simulink model "RL_TTS3_Controller_Blank"  (R2019b)
settings: Solver=FixedStepAuto  StartTime=0.0  StopTime=10.0  FixedStep=0.01  RelTol=1e-3
PostLoadFcn:
  | if any(exist('dsrtsu_mdlpostloadfcn', 'file') ~= 0), dsrtsu_mdlpostloadfcn('Execute', bdroot); end
undefined symbols (not defined in the file or in its folder): Ts
libraries: simulink x2
settings Model: DSRTSU_INTERNAL_RTI_VER=550  DSRTSU_INTERNAL_RTI_TYPE=rti1104  RTICANMMDATA=struct('GeneralSetupData',struct('modelroot','E:\Will\RemoteLabs\TTS3\HostPC','generalsettings',struct('filesettings',struct('destfolder',struct('Name','RTICANMM_FILES','Check',1),'buildfolder',struct('Name','.','Check',1),'AbsDestfolder',struct('Name','E:\Will\RemoteLabs\TTS3\HostPC\RTICANMM_FILES'),'AbsBuildfolder',struct('Name','E:\Will\RemoteLabs\TTS3\HostPC'))),'options',struct('addpaths',1,'rmpaths',1,'addtrcexclusion',true,'cannavigator',struct('checkmonitoring',0),'show_usrtrc',0,'use_usrtrc',0),'advanced',struct('options',ones(1,100)),'MPSetup',{{}},'RTI',struct('Type','RTI1104','Ver','7.13','Date','02-Nov-2019'),'modelname','TTS3_Controller_Test_OL','block','TTS3_Controller_Test_OL'))  DSRTSU_INTERNAL_RTIFPGA=150  Creator=whendrix  LastModifiedBy=edtve
settings DataIOCC: SaveOutput=off  SaveTime=off
settings OptimizationCC: BlockReduction=off  DefaultParameterBehavior=Inlined  OptimizeBlockIOStorage=off  BufferReuse=off  GlobalBufferReuse=off  ExpressionFolding=off  LocalBlockOutputs=off  OptimizeDataStoreBuffers=off  BusAssignmentInplaceUpdate=off
settings DebuggingCC: BusObjectLabelMismatch=none
settings HardwareCC: ProdBitPerPointer=32  ProdBitPerSizeT=32  ProdBitPerPtrDiffT=32  ProdLargestAtomicInteger=Integer  ProdEndianess=BigEndian  ProdWordSize=32  ProdHWDeviceType=Custom Processor->Custom  TargetIntDivRoundTo=Zero  TargetEndianess=BigEndian  TargetHWDeviceType=Custom Processor->Custom
settings ModelReferenceCC: ModelReferenceNumInstancesAllowed=Single  ModelReferenceMinAlgLoopOccurrences=on
settings SFSimCC: MATLABDynamicMemAlloc=off  CustomCodeUndefinedFunction=UseInterfaceOnly
settings RTWCC: Description=dSPACE DS1104 Hardware Platform  SystemTargetFile=rti1104.tlc  MakeCommand=make_rti  TemplateMakefile=rti1104.tmf
settings CodeAppCC: MaxIdLength=63
settings STFCustomTargetCC: ParMdlRefBuildCompliant=on  SystemTargetFile=rti1104.tlc
settings GRTTargetCC: TargetLangStandard=C89/C90 (ANSI)  CompOptLevelCompliant=off  ConcurrentExecutionCompliant=off  CombineOutputUpdateFcns=off  MatFileLogging=off  CPPClassGenCompliant=off  UseToolchainInfoCompliant=off

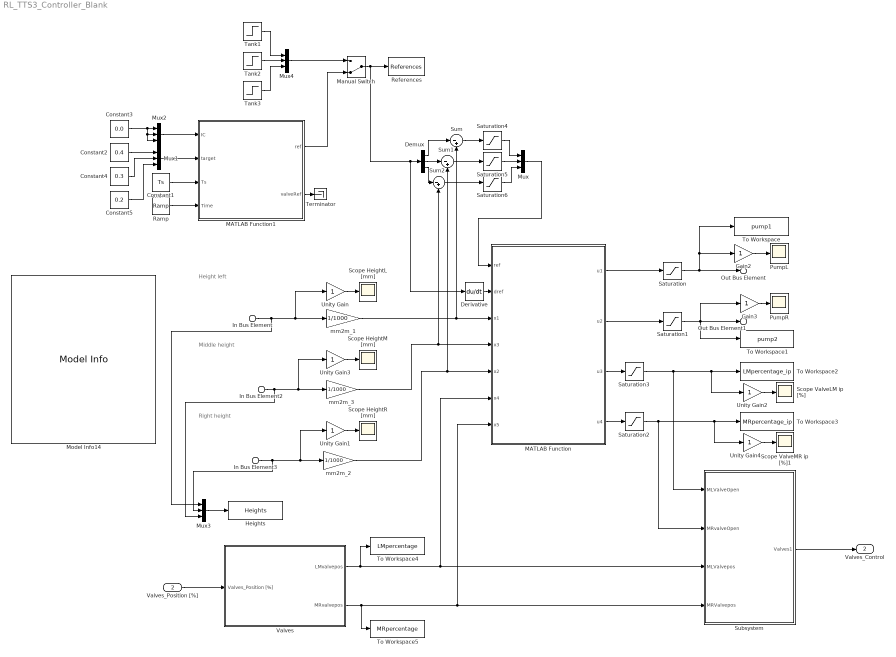
== system RL_TTS3_Controller_Blank ==
  note: Height left
  note: Middle height
  note: Right height
  In Bus Element : Inport  PortName=Heights [mm]  Element=Left
  In Bus Element2 : Inport  PortName=Heights [mm]  Element=Middle
  In Bus Element3 : Inport  PortName=Heights [mm]  Element=Right
  Valves_Position [%] : Inport  Port=2  OutDataTypeStr=Bus: ValvesSOCI
  Constant1 : Constant  Value=Ts
  Constant2 : Constant  Value=0.4
  Constant3 : Constant  Value=0.0
  Constant4 : Constant  Value=0.3
  Constant5 : Constant  Value=0.2
  Demux : Demux  Outputs=3
  Derivative : Derivative
  Gain2 : Gain
  Gain3 : Gain
  Heights : ToWorkspace  VariableName=Heights  SampleTime=-1
  MATLAB Function : MATLAB Function  TreatAsAtomicUnit=on
  MATLAB Function1 : MATLAB Function  TreatAsAtomicUnit=on
  Manual Switch : ManualSwitch  CurrentSetting=0
  Model Info14 : simulink/Model-Wide Utilities/Model Info  Frame=on  DisplayStringWithTags=|  HorizontalTextAlignment=Left  LeftAlignmentValue=0.02
      | Start model for the "Three Tank"
      | experiment on the "Three Tank" setup.
      | Version: 1.0
      | 
      | 
      | INFORMATION
      | ----------------------
      | 
      | Unity Gain block before Scope is needed for
      | RemoteLabs compatebility. 
      | Do not modify or remove!
      | 
      | Pump range:
      | 0 to 0.102 [l/s]
      | 
      | The 5 Valves are labeled according 
      | to their position:
      | 
      |    LM  MR
      |      X     X
      |  X      X      X
      | LD    MD   RD
      | 
      | L = Left
      | M = Middle
      | R = Right
      | D = Down
  Mux{,1..4} (5 alike) : Mux  Inputs=3
  PumpL : Scope
  "PumpR " : Scope
  Ramp : simulink/Sources/Ramp  slope=1  start=0  InitialOutput=0
  "References " : ToWorkspace  VariableName=References  SampleTime=-1
  Saturation : Saturate  UpperLimit=0.1  LowerLimit=0
  Saturation1 : Saturate  UpperLimit=0.1  LowerLimit=0
  Saturation2 : Saturate  UpperLimit=100  LowerLimit=0
  Saturation3 : Saturate  UpperLimit=100  LowerLimit=0
  Saturation4 : Saturate  UpperLimit=1  LowerLimit=-1
  Saturation5 : Saturate  UpperLimit=1  LowerLimit=-1
  Saturation6 : Saturate  UpperLimit=1  LowerLimit=-1
  Scope HeightL [mm] : Scope
  Scope HeightM [mm] : Scope
  Scope HeightR [mm] : Scope
  Scope ValveLM ip [%] : Scope
  Scope ValveMR ip [%]1 : Scope
  Subsystem : Subsystem
  Sum : Sum  Inputs=|-+
  Sum1 : Sum  Inputs=|-+
  Sum2 : Sum  Inputs=|-+
  Tank1 : Step  After=0.3  SampleTime=0
  Tank2 : Step  After=0.3  SampleTime=0
  Tank3 : Step  After=0.3  SampleTime=0
  Terminator : Terminator
  To Workspace : ToWorkspace  VariableName=pump1  SampleTime=-1
  To Workspace1 : ToWorkspace  VariableName=pump2  SampleTime=-1
  To Workspace2 : ToWorkspace  VariableName=LMpercentage_ip  SampleTime=-1
  To Workspace3 : ToWorkspace  VariableName=MRpercentage_ip  SampleTime=-1
  To Workspace4 : ToWorkspace  VariableName=LMpercentage  SampleTime=-1
  To Workspace5 : ToWorkspace  VariableName=MRpercentage  SampleTime=-1
  Unity Gain{,1..4} (5 alike) : Gain
  Valves : Subsystem  TreatAsAtomicUnit=on
  mm2m_1 : Gain  Gain=1/1000
  mm2m_2 : Gain  Gain=1/1000
  mm2m_3 : Gain  Gain=1/1000
  Out Bus Element : Outport  VectorParamsAs1DForOutWhenUnconnected=off  PortName=Pumps [l/s]  Element=Left
  Out Bus Element1 : Outport  VectorParamsAs1DForOutWhenUnconnected=off  PortName=Pumps [l/s]  Element=Right
  Valves_Control : Outport  Port=2  OutDataTypeStr=Bus: ValvesSICO  VectorParamsAs1DForOutWhenUnconnected=off
  wires:
  Unity Gain3/1 -> Scope HeightM [mm]/1
  Unity Gain1/1 -> Scope HeightR [mm]/1
  In Bus Element/1 -> Mux3/1, mm2m_1/1, Unity Gain/1
  In Bus Element2/1 -> Mux3/3, mm2m_3/1, Unity Gain3/1
  Valves_Position [%]/1 -> Valves/1(Valves_Position [%])
  Unity Gain/1 -> Scope HeightL [mm]/1
  Subsystem/1(Valves1) -> Valves_Control/1
  Valves/1(LMvalvepos) -> To Workspace4/1, MATLAB Function/6(x4), Subsystem/3(MLValvepos)
  Valves/2("MRvalvepos ") -> To Workspace5/1, MATLAB Function/7(x5), Subsystem/4(MRValvepos)
  Ramp/1 -> MATLAB Function1/4(Time)
  Constant1/1 -> MATLAB Function1/3(Ts)
  Constant2/1 -> Mux1/1
  Mux1/1 -> MATLAB Function1/2(target)
  Mux2/1 -> MATLAB Function1/1(IC)
  Constant3/1 -> Mux2/3, Mux2/2, Mux2/1
  MATLAB Function1/2(valveRef) -> Terminator/1
  mm2m_1/1 -> Sum/2, MATLAB Function/3(x1)
  mm2m_2/1 -> Sum1/2, MATLAB Function/5(x2)
  mm2m_3/1 -> Sum2/2, MATLAB Function/4(x3)
  MATLAB Function/4(u4) -> Saturation2/1
  MATLAB Function/3(u3) -> Saturation3/1
  Saturation3/1 -> Subsystem/1("MLValveOpen "), Unity Gain2/1, To Workspace2/1
  Saturation2/1 -> Subsystem/2(MRvalveOpen), Unity Gain4/1, To Workspace3/1
  Derivative/1 -> MATLAB Function/2(dref)
  In Bus Element3/1 -> mm2m_2/1, Unity Gain1/1, Mux3/2
  Mux3/1 -> Heights/1
  Tank2/1 -> Mux4/2
  Tank1/1 -> Mux4/1
  Tank3/1 -> Mux4/3
  MATLAB Function1/1(ref) -> Manual Switch/2
  Mux4/1 -> Manual Switch/1
  Manual Switch/1 -> "References "/1, Demux/1, Derivative/1
  Saturation/1 -> To Workspace/1, Gain2/1, Out Bus Element/1
  Saturation1/1 -> To Workspace1/1, Gain3/1, Out Bus Element1/1
  MATLAB Function/2(u2) -> Saturation1/1
  Gain3/1 -> "PumpR "/1
  Gain2/1 -> PumpL/1
  Demux/1 -> Sum/1
  Sum/1 -> Saturation4/1
  Demux/2 -> Sum1/1
  Sum1/1 -> Saturation5/1
  Demux/3 -> Sum2/1
  Sum2/1 -> Saturation6/1
  Saturation5/1 -> Mux/2
  Saturation4/1 -> Mux/1
  Saturation6/1 -> Mux/3
  Mux/1 -> MATLAB Function/1(ref)
  MATLAB Function/1(u1) -> Saturation/1
  Unity Gain2/1 -> Scope ValveLM ip [%]/1
  Unity Gain4/1 -> Scope ValveMR ip [%]1/1
  Constant4/1 -> Mux1/2
  Constant5/1 -> Mux1/3

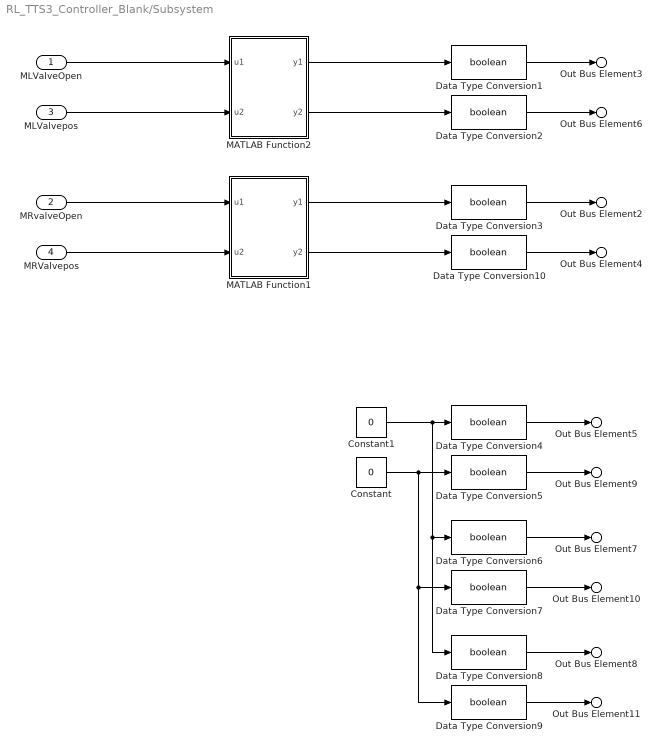
== system RL_TTS3_Controller_Blank/Subsystem ==
  "MLValveOpen " : Inport
  MRvalveOpen : Inport  Port=2
  MLValvepos : Inport  Port=3
  MRValvepos : Inport  Port=4
  Constant : Constant  Value=0
  Constant1 : Constant  Value=0
  Data Type Conversion{1..10} (10 alike) : DataTypeConversion  OutDataTypeStr=boolean
  MATLAB Function1 : MATLAB Function  TreatAsAtomicUnit=on
  MATLAB Function2 : MATLAB Function  TreatAsAtomicUnit=on
  Out Bus Element8 : Outport  VectorParamsAs1DForOutWhenUnconnected=off  PortName=Valves1  Element=RightDown.Open
  Out Bus Element11 : Outport  VectorParamsAs1DForOutWhenUnconnected=off  PortName=Valves1  Element=RightDown.Close
  Out Bus Element5 : Outport  VectorParamsAs1DForOutWhenUnconnected=off  PortName=Valves1  Element=LeftDown.Open
  Out Bus Element9 : Outport  VectorParamsAs1DForOutWhenUnconnected=off  PortName=Valves1  Element=LeftDown.Close
  Out Bus Element7 : Outport  VectorParamsAs1DForOutWhenUnconnected=off  PortName=Valves1  Element=MiddleDown.Open
  Out Bus Element10 : Outport  VectorParamsAs1DForOutWhenUnconnected=off  PortName=Valves1  Element=MiddleDown.Close
  Out Bus Element2 : Outport  VectorParamsAs1DForOutWhenUnconnected=off  PortName=Valves1  Element=MiddleRight.Open
  Out Bus Element4 : Outport  VectorParamsAs1DForOutWhenUnconnected=off  PortName=Valves1  Element=MiddleRight.Close
  Out Bus Element3 : Outport  VectorParamsAs1DForOutWhenUnconnected=off  PortName=Valves1  Element=LeftMiddle.Open
  Out Bus Element6 : Outport  VectorParamsAs1DForOutWhenUnconnected=off  PortName=Valves1  Element=LeftMiddle.Close
  wires:
  Data Type Conversion4/1 -> Out Bus Element5/1
  Data Type Conversion5/1 -> Out Bus Element9/1
  Data Type Conversion8/1 -> Out Bus Element8/1
  Constant1/1 -> Data Type Conversion8/1, Data Type Conversion6/1, Data Type Conversion4/1
  Data Type Conversion9/1 -> Out Bus Element11/1
  Data Type Conversion7/1 -> Out Bus Element10/1
  Data Type Conversion6/1 -> Out Bus Element7/1
  Constant/1 -> Data Type Conversion9/1, Data Type Conversion7/1, Data Type Conversion5/1
  MATLAB Function2/2(y2) -> Data Type Conversion2/1
  MATLAB Function2/1(y1) -> Data Type Conversion1/1
  MATLAB Function1/1(y1) -> Data Type Conversion3/1
  MATLAB Function1/2(y2) -> Data Type Conversion10/1
  MRvalveOpen/1 -> MATLAB Function1/1(u1)
  MRValvepos/1 -> MATLAB Function1/2(u2)
  "MLValveOpen "/1 -> MATLAB Function2/1(u1)
  MLValvepos/1 -> MATLAB Function2/2(u2)
  Data Type Conversion1/1 -> Out Bus Element3/1
  Data Type Conversion2/1 -> Out Bus Element6/1
  Data Type Conversion3/1 -> Out Bus Element2/1
  Data Type Conversion10/1 -> Out Bus Element4/1

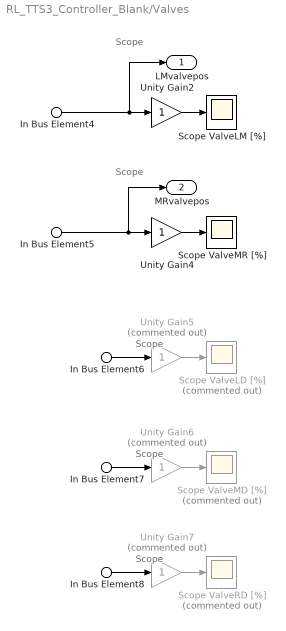
== system RL_TTS3_Controller_Blank/Valves ==
  note: Scope
  note: Scope
  note: Scope
  note: Scope
  note: Scope
  In Bus Element4 : Inport  PortName=Valves_Position [%]  Element=LeftMiddle
  In Bus Element5 : Inport  PortName=Valves_Position [%]  Element=MiddleRight
  In Bus Element6 : Inport  PortName=Valves_Position [%]  Element=LeftDown
  In Bus Element7 : Inport  PortName=Valves_Position [%]  Element=MiddleDown
  In Bus Element8 : Inport  PortName=Valves_Position [%]  Element=RightDown
  Scope ValveLD [%] : Scope  Commented=on
  Scope ValveLM [%] : Scope
  Scope ValveMD [%] : Scope  Commented=on
  Scope ValveMR [%] : Scope
  Scope ValveRD [%] : Scope  Commented=on
  Unity Gain2 : Gain
  Unity Gain4 : Gain
  Unity Gain5 : Gain  Commented=on
  Unity Gain6 : Gain  Commented=on
  Unity Gain7 : Gain  Commented=on
  LMvalvepos : Outport
  "MRvalvepos " : Outport  Port=2
  wires:
  In Bus Element5/1 -> "MRvalvepos "/1, Unity Gain4/1
  In Bus Element4/1 -> Unity Gain2/1, LMvalvepos/1
  In Bus Element7/1 -> Unity Gain6/1
  Unity Gain6/1 -> Scope ValveMD [%]/1
  In Bus Element6/1 -> Unity Gain5/1
  In Bus Element8/1 -> Unity Gain7/1
  Unity Gain7/1 -> Scope ValveRD [%]/1
  Unity Gain4/1 -> Scope ValveMR [%]/1
  Unity Gain5/1 -> Scope ValveLD [%]/1
  Unity Gain2/1 -> Scope ValveLM [%]/1

== matlab function RL_TTS3_Controller_Blank/Subsystem/MATLAB Function2 ==
  data: u1 input; y1 output; y2 output; u2 input
function [y1,y2] = fcn(u1,u2)
    if abs(u1-u2)<=5
        y1 = false;
        y2 = false;
    elseif u2>u1+5
        y1 = false;
        y2 = true;
    elseif u1>u2+5
        y1 = true;
        y2 = false;
    else
        y1 = false;
        y2 = false;
    end
end

== matlab function RL_TTS3_Controller_Blank/MATLAB Function ==
  data: ref input; dref input; x1 input; x3 input; u1 output; u2 output; u3 output; u4 output; x2 input; x4 input; x5 input
%% Sliding mode control for TTS

% Objective 1: independent control of water levels in tank 1 and 2
% Objective 2: keep/move water levels of all tanks on/to one height

% Outputs:     pump1, pump2, valveLM, valveMR
% Inputs:      derivative reference, height tank 1, 2, 3, valveLM, valveMR

function [u1,u2,u3,u4] = SMC_fcn(ref,dref,x1,x3,x2,x4,x5)

option = 2;             % select which control [.]
Atank = 0.0154;         % cross section tanks [m^2]
Sn = 5e-5;              % cross section piper [m^2]
g = 9.81;               % gravity constant [m/s^2]

%% [0] TEST
u1 = 0.05;
u2 = 0.05;
u3 = 0;
u4 = 0;

%% [1] Only control pump 1 and pump 2 (objective 1)
if (option == 1)

    % control objectives (only tanks 1&2)
    s1 = ref(1);
    s2 = ref(2);
    
    % smc vector l and matrix b
    l1  = -1/Atank*Sn*x4/100*sqrt(2*g*abs(x1-x3))-dref(1);
    b11 = 1/Atank;
    l2  = -1/Atank*Sn*x5/100*sqrt(2*g*abs(x2-x3))-dref(2);
    b22 = 1/Atank;
    l = [l1; l2];
    b = [b11, 0; 0, b22];
    
    % controller gains
    k1 = 6;
    k2 = 6;
    
    % controller output
    u  = -inv(b)*(l+[k1*s1; k2*s2]);
    u1 = u(1);
    u2 = u(2);
    u3 = 0.0;
    u4 = 0.0;
    
end
    
%% [2] Control pumps & connecting valves (objective 2)
if (option == 2)
    
    % control objectives (all tanks)
    s1 = ref(1);%x1 - ref(1);
    s2 = ref(2);%x2 - ref(2);
    s3 = ref(3);%x3 - ref(3);
    
    % smc vector l and matrix b
    l1  = -dref(1);
    b11 = 1/Atank;
    b13 = -1/Atank*Sn*1/100*sqrt(2*g*abs(x1-x3));
    l2  = -dref(2);
    b22 = 1/Atank;
    b24 = -1/Atank*Sn*1/100*sqrt(2*g*abs(x2-x3));
    l3  = -dref(3);
    b33 = 1/Atank*Sn*1/100*sqrt(2*g*abs(x1-x3));
    b34 = 1/Atank*Sn*1/100*sqrt(2*g*abs(x2-x3));
    l = [l1; l2; l3];
    b = [b11, 0,   b13, 0; 
         0,   b22, 0,   b24;
         0,   0,   b33, b34];
    
    % controller gains
    k1 = 250;
    k2 = 170;
    k3 = 100;
    
    % controller output
    u  = -pinv(b)*(l+[k1*s1; k2*s2; k3*s3]);
    u1 = u(1);
    u2 = u(2);
    u3 = u(3);
    u4 = u(4);
    
end    

%% [3] Integrator (objective 2)
if (option == 2)
    
    % control objectives (all tanks)
    s1 = ref(1);%x1 - ref(1);
    s2 = ref(2);%x2 - ref(2);
    s3 = ref(3);%x3 - ref(3);
    
    % smc vector l and matrix b
    l1  = -dref(1);
    b11 = 1/Atank;
    b13 = -1/Atank*Sn*1/100*sqrt(2*g*abs(x1-x3));
    l2  = -dref(2);
    b22 = 1/Atank;
    b24 = -1/Atank*Sn*1/100*sqrt(2*g*abs(x2-x3));
    l3  = -dref(3);
    b33 = 1/Atank*Sn*1/100*sqrt(2*g*abs(x1-x3));
    b34 = 1/Atank*Sn*1/100*sqrt(2*g*abs(x2-x3));
    l = [l1; l2; l3];
    b = [b11, 0,   b13, 0; 
         0,   b22, 0,   b24;
         0,   0,   b33, b34];
    
    % controller gains
    k1 = 250;
    k2 = 170;
    k3 = 100;
    K  = [10^-4, 0; 0, 10^-4]; % integral
    
    % controller output
    u  = -pinv(b)*(l+[k1*s1; k2*s2; k3*s3]);
    u1 = u(1);
    u2 = u(2);
    u3 = u(3);
    u4 = u(4);
    
end

== matlab function RL_TTS3_Controller_Blank/Subsystem/MATLAB Function1 ==
  data: u1 input; y1 output; y2 output; u2 input
function [y1,y2] = fcn(u1,u2)
    if abs(u1-u2)<=5
        y1 = false;
        y2 = false;
    elseif u2>u1+5
        y1 = false;
        y2 = true;
    elseif u1>u2+5
        y1 = true;
        y2 = false;
    else
        y1 = false;
        y2 = false;
    end
end

== matlab function RL_TTS3_Controller_Blank/MATLAB Function1 ==
  data: IC input; ref output; target input; valveRef output; Ts input; Time input
function [ref, valveRef] = fcn(IC, target, Ts, Time)
% input: IC, 3D vector of initial conditions of system
% input: target, 3D vector of target reference for fluid  heights
% input: Sampling time Ts

% output: ref, 3*1 vector containing fluid height references [T1 T2 T3]
% output: valveRef, 2*1 vector containg valve references. Needed for MPC,
%         can be ignored (use terminator block in simulink)

%% constants
Atank = 0.0154;
uMaxL = 0.1;        % from Bart's work
uMaxR = 0.09;       % from Bart's work

%% reshaping (check gode generation?)
IC = reshape(IC, [], 1);            %  force IC to be a vector
target = reshape(target, [], 1);    %  idem

%% calculations
tf = 1.1*sum(target)*Atank/(uMaxL+uMaxR-3*0.01)*1000;  % give a 10% margin for pump dynamics etc, choose 50% of maximum disturbance allowed as 'constant disturbance'
ref = zeros(3,1);
valveRef = zeros(2,1);
matr = [1 zeros(1,3);
        0 1  0    0;
        1 tf tf^2 tf^3;
        0 1 2*tf 3*tf^2];
invmatr = inv(matr);
if  Time < tf
    for i =1:3
        vec = [IC(i);0;target(i);0];
        polyCoeff = invmatr*vec;
        ref(i,1) = polyCoeff(1)+polyCoeff(2)*Time+polyCoeff(3)*Time.^2+polyCoeff(4)*Time.^3;
    end
else
    ref = target;
end
